simulink model "PAM_simulink"  (R2013a)
settings: Solver=ode45  StartTime=0.0  StopTime=10.0  RelTol=1e-3
libraries: dsparch4 x2, powerlib_meascontrol x1
settings Model: Creator=lenovo  LastModifiedBy=lenovo

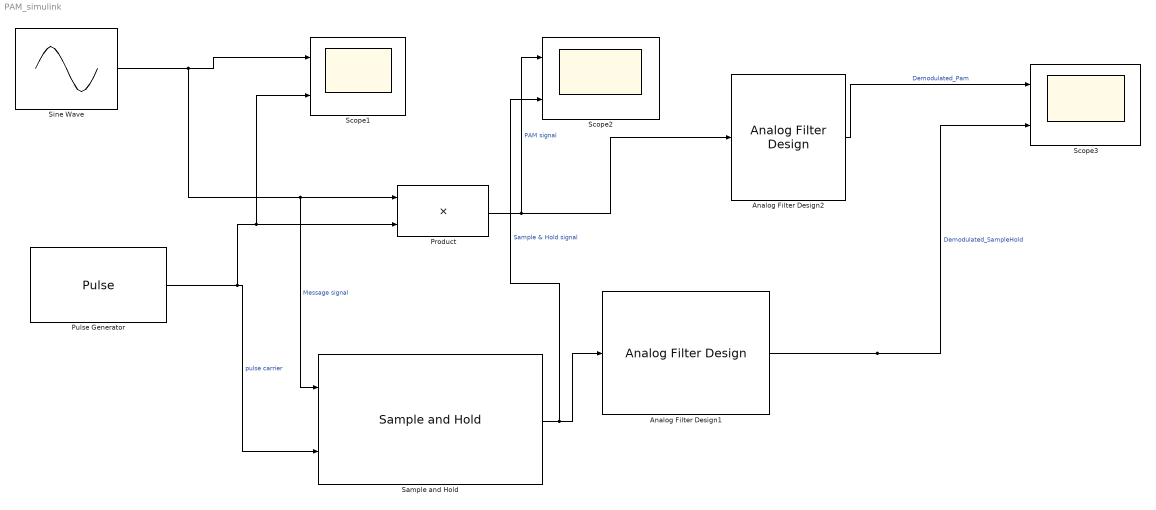
== system PAM_simulink ==
  Analog Filter Design1 : dsparch4/Analog Filter Design  method=Butterworth  filttype=Lowpass  N=7  Wlo=2*pi*10  Whi=80  Rp=2  Rs=40
  Analog Filter Design2 : dsparch4/Analog Filter Design  method=Butterworth  filttype=Lowpass  N=2  Wlo=2*pi*10  Whi=80  Rp=2  Rs=40
  Product : Product
  Pulse Generator : DiscretePulseGenerator  PulseType=Time based  Period=0.02  PulseWidth=50
  Sample and Hold : powerlib_meascontrol/Additional Components/Sample and Hold  ic=0  Ts=0.001
  Scope1 : Scope  NumInputPorts=2
      settings: YMin=-5~-5  YMax=5~5
  Scope2 : Scope  NumInputPorts=2
      settings: YMin=-5~-5  YMax=5~5  SaveName=ScopeData2
  Scope3 : Scope  NumInputPorts=2
      settings: YMin=-5~-5  YMax=5~5
  Sine Wave : Sin  Frequency=2*pi*10  SampleTime=0.001
  wires:
  Sine Wave/1 -> Sample and Hold/1, Product/1, Scope1/1  "Message signal"
  Pulse Generator/1 -> Product/2, Scope1/2, Sample and Hold/2  "pulse carrier"
  Product/1 -> Analog Filter Design2/1, Scope2/1  "PAM signal"
  Sample and Hold/1 -> Analog Filter Design1/1, Scope2/2  "Sample & Hold signal"
  Analog Filter Design2/1 -> Scope3/1  "Demodulated_Pam"
  Analog Filter Design1/1 -> Scope3/2  "Demodulated_SampleHold"
